simulink model "PIcontrolTWOloop"  (Simulink 7.9)
settings: Solver=ode45  StartTime=0.0  StopTime=0.16  FixedStep=1e-6  RelTol=1e-3
libraries: powerlib x15, simulink x1
settings Model: Creator=Administrator  LastModifiedBy=guest1
settings DebuggingCC: StrictBusMsg=Warning
settings CodeAppCC: CustomSymbolStrType=$N$R$M_T
settings GRTTargetCC: CombineOutputUpdateFcns=off  GRTInterface=on

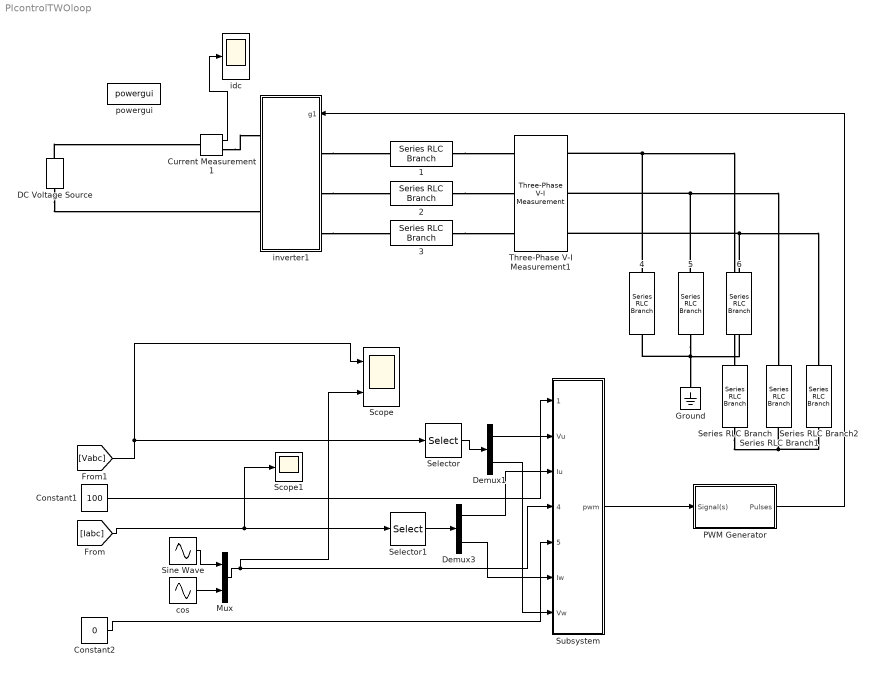
== system PIcontrolTWOloop ==
  1 : powerlib/Elements/Series RLC Branch  LConnTagsString=__new0  RConnTagsString=__new0  BranchType=L  Resistance=1.0  Inductance=2.7e-3  SetiL0=off  InitialCurrent=0  Capacitance=1e-6  Setx0=off  InitialVoltage=0  Measurements=None
  2 : powerlib/Elements/Series RLC Branch  LConnTagsString=__new0  RConnTagsString=__new0  BranchType=L  Resistance=1.0  Inductance=2.7e-3  SetiL0=off  InitialCurrent=0  Capacitance=1e-6  Setx0=off  InitialVoltage=0  Measurements=None
  3 : powerlib/Elements/Series RLC Branch  LConnTagsString=__new0  RConnTagsString=__new0  BranchType=L  Resistance=1.0  Inductance=2.7e-3  SetiL0=off  InitialCurrent=0  Capacitance=1e-6  Setx0=off  InitialVoltage=0  Measurements=None
  4 : powerlib/Elements/Series RLC Branch  LConnTagsString=__new0  RConnTagsString=__new0  BranchType=C  Resistance=0.5  Inductance=8e-3  SetiL0=off  InitialCurrent=0  Capacitance=15e-6  Setx0=off  InitialVoltage=0  Measurements=None
  5 : powerlib/Elements/Series RLC Branch  LConnTagsString=__new0  RConnTagsString=__new0  BranchType=C  Resistance=0.5  Inductance=8e-3  SetiL0=off  InitialCurrent=0  Capacitance=15e-6  Setx0=off  InitialVoltage=0  Measurements=None
  6 : powerlib/Elements/Series RLC Branch  LConnTagsString=__new0  RConnTagsString=__new0  BranchType=C  Resistance=0.5  Inductance=8e-3  SetiL0=off  InitialCurrent=0  Capacitance=15e-6  Setx0=off  InitialVoltage=0  Measurements=None
  Constant1 : Constant  Value=100  OutDataTypeStr=single  SampleTime=1e-4
  Constant2 : Constant  Value=0  OutDataTypeStr=single  SampleTime=1e-4
  Current Measurement1 : powerlib/Measurements/Current Measurement  PhasorSimulation=off  OutputType=Complex  PSBequivalent=0
  DC Voltage Source : powerlib/Electrical Sources/DC Voltage Source  Amplitude=520  Measurements=None
  Demux1 : Demux  Outputs=2
  Demux3 : Demux  Outputs=2
  Ground : powerlib/Elements/Ground  LConnTagsString=a
  Mux : Mux  Inputs=2
  PWM Generator : Subsystem  AncestorBlock="powerlib_extras/Control  Blocks/PWM Generator"  DialogController=POWERSYS.PowerSysDialog  mask(PWM Generator){GeneratorMode=3-arm  bridge (6 pulses), Fc=10000, Internal=off, mIndex=0.4, Freq=60, Phase=0}
      mask prompts: GeneratorMode "Generator Mode"; Fc "Carrier frequency (Hz):"; Internal "Internal generation of modulating signal(s)"; mIndex "Modulation index  (0<m<1) :"; Freq "Frequency of output voltage (Hz)"; Phase "Phase of output voltage (degrees)"
      mask help:
      | This block generates pulses for carrier-based PWM (Pulse Width Modulation), self-commutated IGBTs,GTOs or FETs bridges.
      |
      | Depending on the number of bridge arms selected in the "Generator Mode" parameter, the block can be used either for single-phase or three-phase PWM control.
      mask init:
      | powericon('psbcallbacks',gcb,'PWM Generator');
      | if Freq==0
      |     Phase=90;
      | end
      | switch GeneratorMode
      | case 1,
      |     Internal_Phase=0;
      |    Signal_PortWidth=1;
      |    Select1_Elements=[1 2];
      |    Select1_PortWidth=2;
      |    Select3_Elements=[1 2];
      |    Select3_PortWidth=4;
      | case 2,
      |     Internal_Phase=0;
      |     Signal_PortWidth=1;
      |     Select1_Elements=[1 2];
      |     Select1_PortWidth=2;
      |     Select3_Elements=[1 2 3 4];
      |     Select3_PortWidth=4;
      | case 3,
      |     Internal_Phase=[0 -2*pi/3 2*pi/3];
      |     Signal_PortWidth=3;
      |     Select1_Elements=[1 4 2 5 3 6];
      |     Select1_PortWidth=6;
      |    Select3_Elements=[1 2 3 4 5 6];
      |    Select3_PortWidth=12;
      | case 4,
      |     Internal_Phase=[0 -2*pi/3 2*pi/3];
      |     Signal_PortWidth=3;
      |     Select1_Elements=[1 4 2 5 3 6];
      |     Select1_PortWidth=6;
      |    Select3_Elements=[1 2 3 4 5 6 7 8 9 10 11 12];
      |    Select3_PortWidth=12;
      | end
      | power_initmask();
      mask Help: web(psbhelp)
      mask StyleString: popup(1-arm  bridge (2 pulses)|2-arm  bridge (4 pulses)|3-arm  bridge (6 pulses)|Double 3-arm  bridges (12 pulses)),edit,checkbox,edit,edit,edit
      mask Display: disp('')
  Scope : Scope  NumInputPorts=2
      settings: TimeRange=0.1  YMin=-110~-1.25  YMax=110~1.25
  Scope1 : Scope
      settings: TimeRange=0.1  YMin=-1.75  YMax=1.5
  Selector : Selector  InputPortWidth=3  IndexOptions=Index vector (dialog)  Indices=[1 3]  OutputSizes=1
  Selector1 : Selector  InputPortWidth=3  IndexOptions=Index vector (dialog)  Indices=[1 3]  OutputSizes=1
  Series RLC Branch : powerlib/Elements/Series RLC Branch  LConnTagsString=__new0  RConnTagsString=__new0  BranchType=R  Resistance=12  Inductance=1e-3  SetiL0=off  InitialCurrent=0  Capacitance=1e-6  Setx0=off  InitialVoltage=0  Measurements=None
  Series RLC Branch1 : powerlib/Elements/Series RLC Branch  LConnTagsString=__new0  RConnTagsString=__new0  BranchType=R  Resistance=12  Inductance=1e-3  SetiL0=off  InitialCurrent=0  Capacitance=1e-6  Setx0=off  InitialVoltage=0  Measurements=None
  Series RLC Branch2 : powerlib/Elements/Series RLC Branch  LConnTagsString=__new0  RConnTagsString=__new0  BranchType=R  Resistance=12  Inductance=1e-3  SetiL0=off  InitialCurrent=0  Capacitance=1e-6  Setx0=off  InitialVoltage=0  Measurements=None
  Sine Wave : Sin  Frequency=2*pi*50  SampleTime=1e-4
  Subsystem : Subsystem
  Three-Phase V-I Measurement1 : powerlib/Measurements/Three-Phase V-I Measurement  VoltageMeasurement=phase-to-ground  SetLabelV=on  LabelV=Vabc  Vpu=off  VpuLL=off  CurrentMeasurement=yes  SetLabelI=on  LabelI=Iabc  Ipu=off  Pbase=100e6  Vbase=500e3  OutputType=Complex  PhasorSimulation=off  PSBequivalent=0
  cos : Sin  Frequency=2*pi*50  Phase=pi/2  SampleTime=1e-4
  idc : Scope
      settings: TimeRange=1  YMin=0  YMax=9.5  SaveName=idc
  inverter1 : Subsystem
  powergui : powerlib/powergui  SimulationMode=Discrete  SolverType=Tustin  SampleTime=1e-7  frequency=60  SPID=on  DisableSnubberDevices=off  DisableRonSwitches=off  DisableVfSwitches=off  SwTol=0  Interpol=off  DisplayEquations=off  FunctionMessages=off  frequencyindice=0  Pbase=100e6  ErrMax=1e-4  Iterations=50  UnitsV=kV  UnitsW=MW  echomessages=off  HookPort=off  EnableUseOfTLC=off  x0status=blocks  RestoreLinks=warning  ResistiveCurrentMeasurement=off  Frange=[0:2:500]  Ylog=off  Xlog=on  ShowGrid=off  save=off  variable=ZData  structure=ScopeData  ZoomFFT=off  StartTime=0.04  cycles=2  DisplayStyle=2  fundamental=50  FreqAxis=on  MaxFrequency=120000  frequencyindicesteady=1  RmsSteady=1  display=off  Ts=0  methode=off
  wires:
  Current Measurement1/1 -> idc/1
  Sine Wave/1 -> Mux/1
  cos/1 -> Mux/2
  Constant1/1 -> Subsystem/1(Vd_ref)
  Constant2/1 -> Subsystem/5(Vq_ref)
  Mux/1 -> Scope/2, Subsystem/4(sincos)
  [Iabc] -> Scope1/1, Selector1/1
  [Vabc] -> Scope/1, Selector/1
  Selector/1 -> Demux1/1
  Selector1/1 -> Demux3/1
  Demux1/1 -> Subsystem/2(Vu)
  Demux1/2 -> Subsystem/7(Vw)
  Demux3/1 -> Subsystem/3(Iu)
  Demux3/2 -> Subsystem/6(Iw)
  Subsystem/1(pwm) -> PWM Generator/1(Signal(s))
  PWM Generator/1(Pulses) -> inverter1/1(g1)
  connections:
  4/RConn1 -- 5/RConn1 -- 6/RConn1 -- Ground/LConn1
  4/LConn1 -- Three-Phase V-I Measurement1/RConn1 -- Series RLC Branch/LConn1
  5/LConn1 -- Three-Phase V-I Measurement1/RConn2 -- Series RLC Branch1/LConn1
  6/LConn1 -- Three-Phase V-I Measurement1/RConn3 -- Series RLC Branch2/LConn1
  DC Voltage Source/RConn1 -- Current Measurement1/LConn1
  inverter1/LConn3 -- 3/LConn1
  inverter1/LConn2 -- 2/LConn1
  inverter1/LConn1 -- 1/LConn1
  DC Voltage Source/LConn1 -- inverter1/RConn2
  1/RConn1 -- Three-Phase V-I Measurement1/LConn1
  3/RConn1 -- Three-Phase V-I Measurement1/LConn3
  2/RConn1 -- Three-Phase V-I Measurement1/LConn2
  Current Measurement1/RConn1 -- inverter1/RConn1
  Series RLC Branch2/RConn1 -- Series RLC Branch/RConn1 -- Series RLC Branch1/RConn1

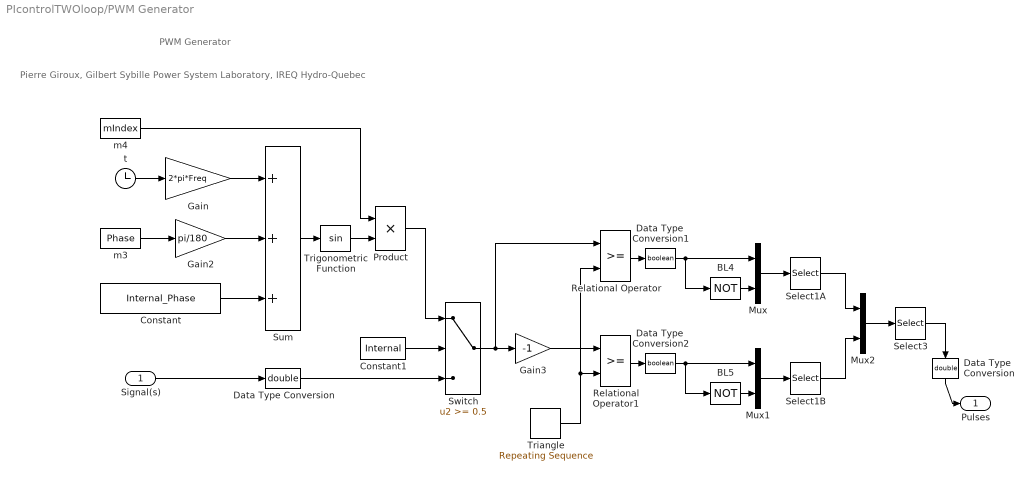
== system PIcontrolTWOloop/PWM Generator ==
  note: PWM Generator
  note: Pierre Giroux, Gilbert Sybille
      | Power System Laboratory, IREQ
      | Hydro-Quebec
  Signal(s) : Inport
  BL4 : Logic  Operator=NOT  Inputs=1
  BL5 : Logic  Operator=NOT  Inputs=1
  Constant : Constant  Value=Internal_Phase
  Constant1 : Constant  Value=Internal
  Data Type  Conversion : DataTypeConversion  OutDataTypeStr=double  SaturateOnIntegerOverflow=on  RndMeth=Zero
  Data Type  Conversion1 : DataTypeConversion  OutDataTypeStr=boolean  SaturateOnIntegerOverflow=on  RndMeth=Zero
  Data Type  Conversion2 : DataTypeConversion  OutDataTypeStr=boolean  SaturateOnIntegerOverflow=on  RndMeth=Zero
  Data Type Conversion : DataTypeConversion  OutDataTypeStr=double
  Gain : Gain  Gain=2*pi*Freq  SaturateOnIntegerOverflow=on  OutDataTypeStr=Inherit: Same as input  ParamDataTypeStr=Inherit: Same as input
  Gain2 : Gain  Gain=pi/180  SaturateOnIntegerOverflow=on  OutDataTypeStr=Inherit: Same as input  ParamDataTypeStr=Inherit: Same as input
  Gain3 : Gain  Gain=-1  SaturateOnIntegerOverflow=on  OutDataTypeStr=Inherit: Same as input  ParamDataTypeStr=Inherit: Same as input
  Mux : Mux  Inputs=2
  Mux1 : Mux  Inputs=2
  Mux2 : Mux  Inputs=2
  Product : Product  SaturateOnIntegerOverflow=on  InputSameDT=on  OutDataTypeStr=Inherit: Same as first input
  Relational Operator : RelationalOperator  InputSameDT=on
  Relational Operator1 : RelationalOperator  InputSameDT=on
  Select1A : Selector  InputPortWidth=Select1_PortWidth  IndexOptions=Index vector (dialog)  Indices=Select1_Elements  OutputSizes=1
  Select1B : Selector  InputPortWidth=Select1_PortWidth  IndexOptions=Index vector (dialog)  Indices=Select1_Elements  OutputSizes=1
  Select3 : Selector  InputPortWidth=Select3_PortWidth  IndexOptions=Index vector (dialog)  Indices=Select3_Elements  OutputSizes=1
  Sum : Sum  Inputs=+++  SaturateOnIntegerOverflow=on  InputSameDT=on  OutDataTypeStr=Inherit: Same as first input
  Switch : Switch  Threshold=0.5  InputSameDT=on
  Triangle : simulink/Sources/Repeating Sequence  rep_seq_t=[0 1/Fc/4 3/Fc/4 1/Fc]  rep_seq_y=[0 -260 260 0]
  Trigonometric Function : Trigonometry
  m3 : Constant  Value=Phase
  m4 : Constant  Value=mIndex
  t : Clock
  Pulses : Outport
  wires:
  Data Type  Conversion2/1 -> Mux1/1, BL5/1
  Relational Operator1/1 -> Data Type  Conversion2/1
  Data Type  Conversion1/1 -> Mux/1, BL4/1
  Relational Operator/1 -> Data Type  Conversion1/1
  Data Type  Conversion/1 -> Pulses/1
  Select3/1 -> Data Type  Conversion/1
  t/1 -> Gain/1
  Gain/1 -> Sum/1
  Gain2/1 -> Sum/2
  m3/1 -> Gain2/1
  Constant/1 -> Sum/3
  m4/1 -> Product/1
  Sum/1 -> Trigonometric Function/1
  Trigonometric Function/1 -> Product/2
  Signal(s)/1 -> Data Type Conversion/1
  Constant1/1 -> Switch/2
  Product/1 -> Switch/1
  Gain3/1 -> Relational Operator1/1
  BL4/1 -> Mux/2
  BL5/1 -> Mux1/2
  Mux/1 -> Select1A/1
  Mux1/1 -> Select1B/1
  Select1A/1 -> Mux2/1
  Select1B/1 -> Mux2/2
  Mux2/1 -> Select3/1
  Switch/1 -> Gain3/1, Relational Operator/1
  Triangle/1 -> Relational Operator1/2, Relational Operator/2
  Data Type Conversion/1 -> Switch/3

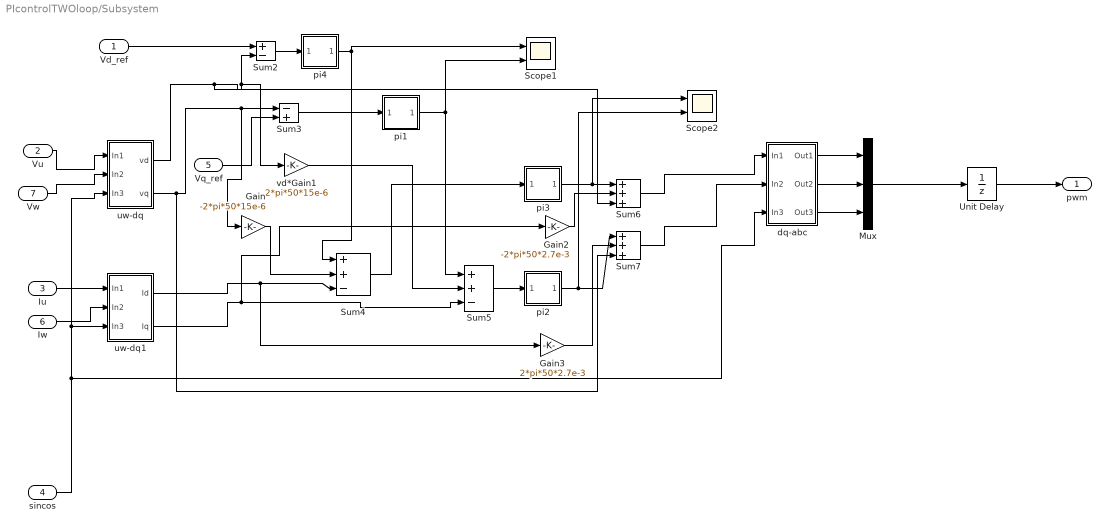
== system PIcontrolTWOloop/Subsystem ==
  Vd_ref : Inport
  Vu : Inport  Port=2
  Iu : Inport  Port=3
  sincos : Inport  Port=4
  Vq_ref : Inport  Port=5
  Iw : Inport  Port=6
  Vw : Inport  Port=7
  Gain : Gain  Gain=-2*pi*50*15e-6
  Gain2 : Gain  Gain=-2*pi*50*2.7e-3
  Gain3 : Gain  Gain=2*pi*50*2.7e-3
  Mux : Mux  Inputs=3
  Scope1 : Scope  NumInputPorts=2
      settings: TimeRange=0.1  YMin=62~0.2  YMax=78~1.7  SaveName=ScopeData2
  Scope2 : Scope  NumInputPorts=2
      settings: TimeRange=0.1  YMin=-17.5~-5  YMax=15~5  SaveName=ScopeData3
  Sum2 : Sum  Inputs=+-
  Sum3 : Sum  Inputs=-+
  Sum4 : Sum  Inputs=++-
  Sum5 : Sum  Inputs=++-
  Sum6 : Sum  Inputs=+++
  Sum7 : Sum  Inputs=+++
  Unit Delay : UnitDelay  SampleTime=-1
  dq-abc : Subsystem
  pi1 : Subsystem
  pi2 : Subsystem
  pi3 : Subsystem
  pi4 : Subsystem
  uw-dq : Subsystem
  uw-dq1 : Subsystem
  vd*Gain1 : Gain  Gain=2*pi*50*15e-6
  pwm : Outport
  wires:
  vd*Gain1/1 -> Sum5/2
  Gain/1 -> Sum4/2
  Gain2/1 -> Sum6/2
  Gain3/1 -> Sum7/2
  Sum7/1 -> dq-abc/2(In2)
  Sum6/1 -> dq-abc/1(In1)
  pi2/1(Out1) -> Sum7/1, Scope2/2
  pi3/1(Out1) -> Sum6/1, Scope2/1
  uw-dq1/1(Id) -> Sum4/3, Gain3/1
  uw-dq1/2(Iq) -> Sum5/3, Gain2/1
  Sum5/1 -> pi2/1(In1)
  pi1/1(Out1) -> Sum5/1, Scope1/2
  Sum4/1 -> pi3/1(In1)
  pi4/1(Out1) -> Sum4/1, Scope1/1
  Sum3/1 -> pi1/1(In1)
  Vq_ref/1 -> Sum3/2
  Sum2/1 -> pi4/1(In1)
  Vd_ref/1 -> Sum2/1
  sincos/1 -> uw-dq/3(In3), uw-dq1/3(In3), dq-abc/3(In3)
  Vu/1 -> uw-dq/1(In1)
  Iu/1 -> uw-dq1/1(In1)
  Vw/1 -> uw-dq/2(In2)
  uw-dq/1(vd) -> Sum6/3, Sum2/2, vd*Gain1/1
  uw-dq/2(vq) -> Sum7/3, Sum3/1, Gain/1
  Iw/1 -> uw-dq1/2(In2)
  dq-abc/1(Out1) -> Mux/1
  dq-abc/2(Out2) -> Mux/2
  dq-abc/3(Out3) -> Mux/3
  Mux/1 -> Unit Delay/1
  Unit Delay/1 -> pwm/1

== system PIcontrolTWOloop/inverter1 ==
  g1 : Inport
  Universal Bridge : powerlib/Power Electronics/Universal Bridge  Arms=3  SnubberResistance=5000  SnubberCapacitance=inf  Device=IGBT / Diodes  Ron=1e-3  Lon=0  ForwardVoltages="[  0  0  ]"  ForwardVoltage=0  GTOparameters=[ 10e-6 , 20e-6 ]  IGBTparameters=[ 1e-6 , 2e-6 ]  Measurements=All voltages and currents  Measurements_2=None  converterType=Rectifier
  A : PMIOPort  Port=1  Side=Left
  B : PMIOPort  Port=2  Side=Left
  C : PMIOPort  Port=3  Side=Left
  Vdc1 : PMIOPort  Port=4  Side=Right
  Vdc2 : PMIOPort  Port=5  Side=Right
  wires:
  g1/1 -> Universal Bridge/1
  connections:
  Universal Bridge/RConn1 -- Vdc1/RConn1
  Universal Bridge/RConn2 -- Vdc2/RConn1
  Universal Bridge/LConn1 -- A/RConn1
  Universal Bridge/LConn2 -- B/RConn1
  Universal Bridge/LConn3 -- C/RConn1

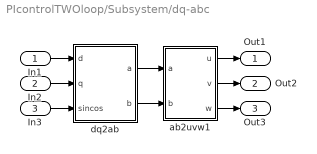
== system PIcontrolTWOloop/Subsystem/dq-abc ==
  In1 : Inport
  In2 : Inport  Port=2
  In3 : Inport  Port=3
  ab2uvw1 : Subsystem
  dq2ab : Subsystem
  Out1 : Outport
  Out2 : Outport  Port=2
  Out3 : Outport  Port=3
  wires:
  dq2ab/1(a) -> ab2uvw1/1(a)
  dq2ab/2(b) -> ab2uvw1/2(b)
  ab2uvw1/1(u) -> Out1/1
  In1/1 -> dq2ab/1(d)
  ab2uvw1/2(v) -> Out2/1
  In2/1 -> dq2ab/2(q)
  ab2uvw1/3(w) -> Out3/1
  In3/1 -> dq2ab/3(sincos)

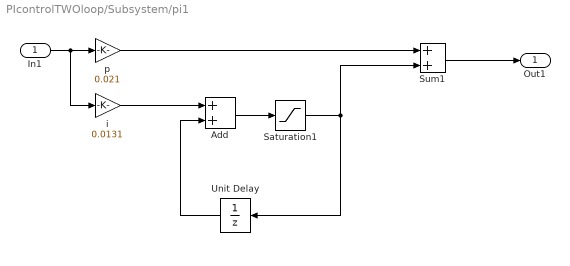
== system PIcontrolTWOloop/Subsystem/pi1 ==
  In1 : Inport
  Add : Sum  AccumDataTypeStr=single  OutDataTypeStr=single  RndMeth=Nearest
  Saturation1 : Saturate  UpperLimit=20  LowerLimit=-20  LinearizeAsGain=off  ZeroCross=off
  Sum1 : Sum
  Unit Delay : UnitDelay  SampleTime=1e-4
  i : Gain  Gain=0.0131  OutDataTypeStr=single  RndMeth=Nearest
  p : Gain  Gain=0.021  OutDataTypeStr=single  RndMeth=Nearest
  Out1 : Outport
  wires:
  Saturation1/1 -> Unit Delay/1, Sum1/2
  p/1 -> Sum1/1
  Sum1/1 -> Out1/1
  Unit Delay/1 -> Add/2
  Add/1 -> Saturation1/1
  i/1 -> Add/1
  In1/1 -> i/1, p/1

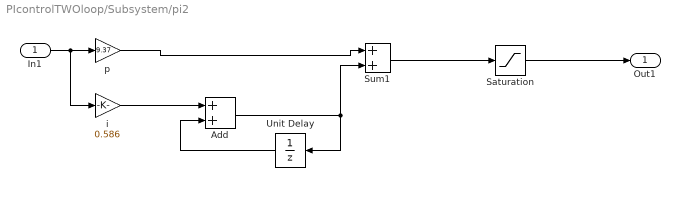
== system PIcontrolTWOloop/Subsystem/pi2 ==
  In1 : Inport
  Add : Sum  AccumDataTypeStr=single  OutDataTypeStr=single  RndMeth=Nearest
  Saturation : Saturate  UpperLimit=300  LowerLimit=-300  LinearizeAsGain=off  ZeroCross=off
  Sum1 : Sum
  Unit Delay : UnitDelay  SampleTime=1e-4
  i : Gain  Gain=0.586  OutDataTypeStr=single  RndMeth=Nearest
  p : Gain  Gain=9.37  OutDataTypeStr=single  RndMeth=Nearest
  Out1 : Outport
  wires:
  p/1 -> Sum1/1
  Saturation/1 -> Out1/1
  Sum1/1 -> Saturation/1
  Unit Delay/1 -> Add/2
  Add/1 -> Unit Delay/1, Sum1/2
  i/1 -> Add/1
  In1/1 -> i/1, p/1

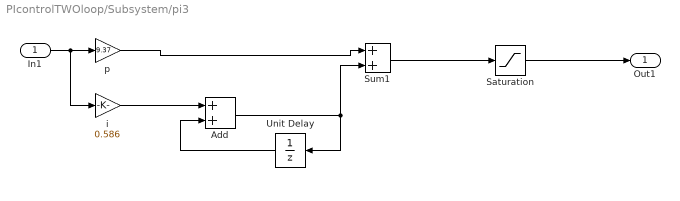
== system PIcontrolTWOloop/Subsystem/pi3 ==
  In1 : Inport
  Add : Sum  AccumDataTypeStr=single  OutDataTypeStr=single  RndMeth=Nearest
  Saturation : Saturate  UpperLimit=300  LowerLimit=-300  LinearizeAsGain=off  ZeroCross=off
  Sum1 : Sum
  Unit Delay : UnitDelay  SampleTime=1e-4
  i : Gain  Gain=0.586  OutDataTypeStr=single  RndMeth=Nearest
  p : Gain  Gain=9.37  OutDataTypeStr=single  RndMeth=Nearest
  Out1 : Outport
  wires:
  In1/1 -> p/1, i/1
  i/1 -> Add/1
  Add/1 -> Sum1/2, Unit Delay/1
  Unit Delay/1 -> Add/2
  Sum1/1 -> Saturation/1
  Saturation/1 -> Out1/1
  p/1 -> Sum1/1

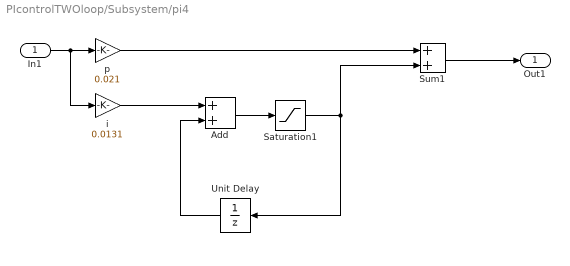
== system PIcontrolTWOloop/Subsystem/pi4 ==
  In1 : Inport
  Add : Sum  AccumDataTypeStr=single  OutDataTypeStr=single  RndMeth=Nearest
  Saturation1 : Saturate  UpperLimit=20  LowerLimit=-20  LinearizeAsGain=off  ZeroCross=off
  Sum1 : Sum
  Unit Delay : UnitDelay  SampleTime=1e-4
  i : Gain  Gain=0.0131  OutDataTypeStr=single  RndMeth=Nearest
  p : Gain  Gain=0.021  OutDataTypeStr=single  RndMeth=Nearest
  Out1 : Outport
  wires:
  In1/1 -> p/1, i/1
  i/1 -> Add/1
  Add/1 -> Saturation1/1
  Unit Delay/1 -> Add/2
  Sum1/1 -> Out1/1
  p/1 -> Sum1/1
  Saturation1/1 -> Sum1/2, Unit Delay/1

== system PIcontrolTWOloop/Subsystem/uw-dq ==
  In1 : Inport
  In2 : Inport  Port=2
  In3 : Inport  Port=3
  ab2dq : Subsystem
  uw2ab4 : Subsystem
  vd : Outport
  vq : Outport  Port=2
  wires:
  uw2ab4/2(b) -> ab2dq/2(b)
  uw2ab4/1(a) -> ab2dq/1(a)
  In1/1 -> uw2ab4/1(u)
  ab2dq/1(d) -> vd/1
  In2/1 -> uw2ab4/2(w)
  ab2dq/2(q) -> vq/1
  In3/1 -> ab2dq/3(sincos)

== system PIcontrolTWOloop/Subsystem/uw-dq1 ==
  In1 : Inport
  In2 : Inport  Port=2
  In3 : Inport  Port=3
  ab2dq : Subsystem
  uw2ab4 : Subsystem
  Id : Outport
  Iq : Outport  Port=2
  wires:
  uw2ab4/2(b) -> ab2dq/2(b)
  uw2ab4/1(a) -> ab2dq/1(a)
  In1/1 -> uw2ab4/1(u)
  ab2dq/1(d) -> Id/1
  In2/1 -> uw2ab4/2(w)
  ab2dq/2(q) -> Iq/1
  In3/1 -> ab2dq/3(sincos)

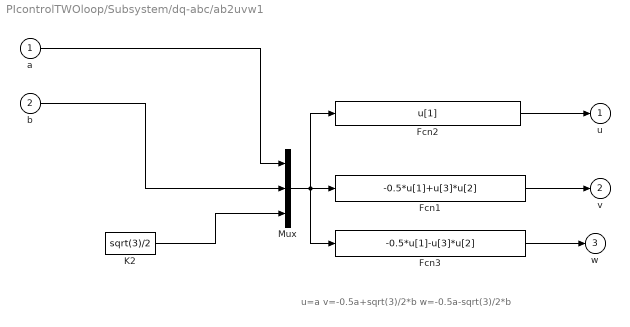
== system PIcontrolTWOloop/Subsystem/dq-abc/ab2uvw1 ==
  note: u=a
      | v=-0.5a+sqrt(3)/2*b
      | w=-0.5a-sqrt(3)/2*b
  a : Inport  OutDataTypeStr=double  PortDimensions=1
  b : Inport  Port=2  OutDataTypeStr=double  PortDimensions=1
  Fcn1 : Fcn  Expr=-0.5*u[1]+u[3]*u[2]
  Fcn2 : Fcn  Expr=u[1]
  Fcn3 : Fcn  Expr=-0.5*u[1]-u[3]*u[2]
  K2 : Constant  Value=sqrt(3)/2  OutDataTypeStr=double
  Mux : Mux  Inputs=3
  u : Outport  InitialOutput=0
  v : Outport  Port=2  InitialOutput=0
  w : Outport  Port=3  InitialOutput=0
  wires:
  Mux/1 -> Fcn1/1, Fcn2/1, Fcn3/1
  a/1 -> Mux/1
  K2/1 -> Mux/3
  b/1 -> Mux/2
  Fcn1/1 -> v/1
  Fcn2/1 -> u/1
  Fcn3/1 -> w/1

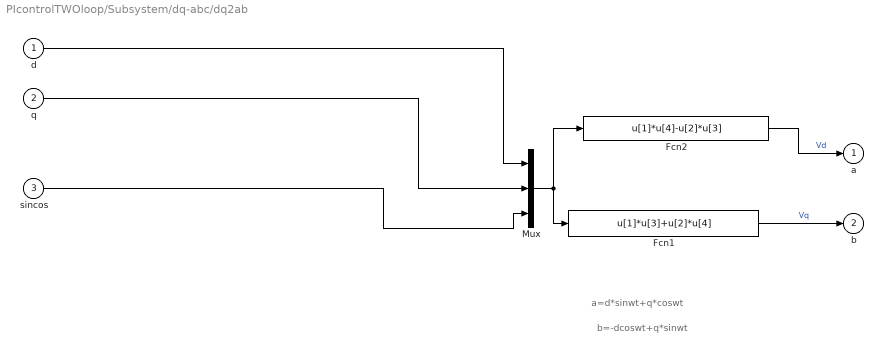
== system PIcontrolTWOloop/Subsystem/dq-abc/dq2ab ==
  note: a=d*sinwt+q*coswt
  note: b=-dcoswt+q*sinwt
  d : Inport  PortDimensions=1
  q : Inport  Port=2  PortDimensions=1
  sincos : Inport  Port=3  PortDimensions=2
  Fcn1 : Fcn  Expr=u[1]*u[3]+u[2]*u[4]
  Fcn2 : Fcn  Expr=u[1]*u[4]-u[2]*u[3]
  Mux : Mux  Inputs=3
  a : Outport  InitialOutput=0
  b : Outport  Port=2  InitialOutput=0
  wires:
  Mux/1 -> Fcn1/1, Fcn2/1
  d/1 -> Mux/1
  q/1 -> Mux/2
  sincos/1 -> Mux/3
  Fcn2/1 -> a/1  "Vd"
  Fcn1/1 -> b/1  "Vq"

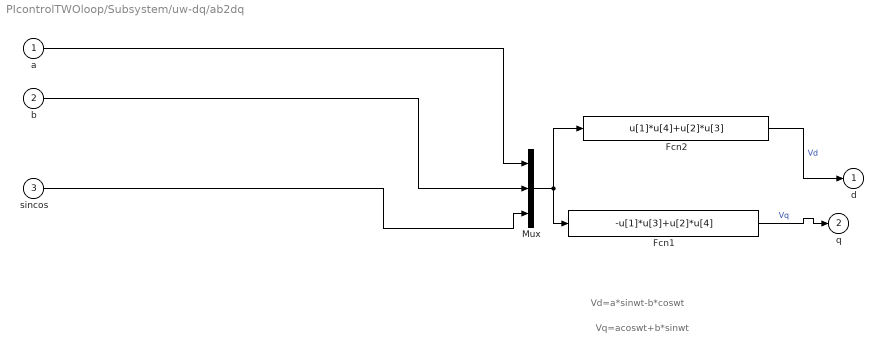
== system PIcontrolTWOloop/Subsystem/uw-dq/ab2dq ==
  note: Vd=a*sinwt-b*coswt
  note: Vq=acoswt+b*sinwt
  a : Inport  PortDimensions=1
  b : Inport  Port=2  PortDimensions=1
  sincos : Inport  Port=3  PortDimensions=2
  Fcn1 : Fcn  Expr=-u[1]*u[3]+u[2]*u[4]
  Fcn2 : Fcn  Expr=u[1]*u[4]+u[2]*u[3]
  Mux : Mux  Inputs=3
  d : Outport  InitialOutput=0
  q : Outport  Port=2  InitialOutput=0
  wires:
  Fcn2/1 -> d/1  "Vd"
  Fcn1/1 -> q/1  "Vq"
  Mux/1 -> Fcn1/1, Fcn2/1
  a/1 -> Mux/1
  b/1 -> Mux/2
  sincos/1 -> Mux/3

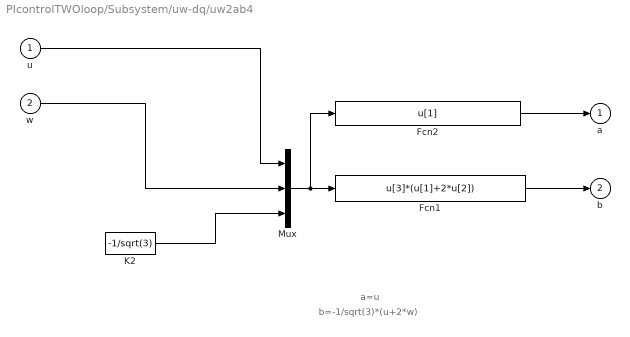
== system PIcontrolTWOloop/Subsystem/uw-dq/uw2ab4 ==
  note: a=u
  note: b=-1/sqrt(3)*(u+2*w)
  u : Inport  PortDimensions=1
  w : Inport  Port=2  PortDimensions=1
  Fcn1 : Fcn  Expr=u[3]*(u[1]+2*u[2])
  Fcn2 : Fcn  Expr=u[1]
  K2 : Constant  Value=-1/sqrt(3)  OutDataTypeStr=double
  Mux : Mux  Inputs=3
  a : Outport  InitialOutput=0
  b : Outport  Port=2  InitialOutput=0
  wires:
  Mux/1 -> Fcn1/1, Fcn2/1
  u/1 -> Mux/1
  K2/1 -> Mux/3
  w/1 -> Mux/2
  Fcn1/1 -> b/1
  Fcn2/1 -> a/1

== system PIcontrolTWOloop/Subsystem/uw-dq1/ab2dq ==
  note: Vd=a*sinwt-b*coswt
  note: Vq=acoswt+b*sinwt
  a : Inport  PortDimensions=1
  b : Inport  Port=2  PortDimensions=1
  sincos : Inport  Port=3  PortDimensions=2
  Fcn1 : Fcn  Expr=-u[1]*u[3]+u[2]*u[4]
  Fcn2 : Fcn  Expr=u[1]*u[4]+u[2]*u[3]
  Mux : Mux  Inputs=3
  d : Outport  InitialOutput=0
  q : Outport  Port=2  InitialOutput=0
  wires:
  Fcn2/1 -> d/1  "Vd"
  Fcn1/1 -> q/1  "Vq"
  Mux/1 -> Fcn1/1, Fcn2/1
  a/1 -> Mux/1
  b/1 -> Mux/2
  sincos/1 -> Mux/3

== system PIcontrolTWOloop/Subsystem/uw-dq1/uw2ab4 ==
  note: a=u
  note: b=-1/sqrt(3)*(u+2*w)
  u : Inport  PortDimensions=1
  w : Inport  Port=2  PortDimensions=1
  Fcn1 : Fcn  Expr=u[3]*(u[1]+2*u[2])
  Fcn2 : Fcn  Expr=u[1]
  K2 : Constant  Value=-1/sqrt(3)  OutDataTypeStr=double
  Mux : Mux  Inputs=3
  a : Outport  InitialOutput=0
  b : Outport  Port=2  InitialOutput=0
  wires:
  Mux/1 -> Fcn1/1, Fcn2/1
  u/1 -> Mux/1
  K2/1 -> Mux/3
  w/1 -> Mux/2
  Fcn1/1 -> b/1
  Fcn2/1 -> a/1
